simulink model "LQR_v9_two_separate_gyros_discrete"  (R2017b)
settings: Solver=VariableStepAuto  StartTime=0.0  StopTime=10  FixedStep=0.005  RelTol=1e-3
values from neighbouring files (symbols this model uses):
  A = [0 0 0 1 0 0 ... (first row only)    [LQR_PLACE_v9_sep_gryos.m]
  B = [0 0 ... (first row only)    [LQR_PLACE_v9_sep_gryos.m]
  C = [1 0 0 0 0 0 ... (first row only)    [LQR_PLACE_v9_sep_gryos.m]
  Dist_period = 10    [LQR_PLACE_v9_sep_gryos.m]
  F_d = 0    [LQR_PLACE_v9_sep_gryos.m]
  Fd = 300    [LQR_PLACE_v9_sep_gryos.m]
  Init_cond = [ roll_angle, precession_angle1, precession_angle2, roll_rate,     precession_rate1, precession_rate2 ]    [LQR_PLACE_v9_sep_gryos.m]
  Ts = Ts_min    [LQR_PLACE_v9_sep_gryos.m]
  V = [0 ... (first row only)    [LQR_PLACE_v9_sep_gryos.m]
  W = [0 ... (first row only)    [LQR_PLACE_v9_sep_gryos.m]
undefined symbols (not defined in the file or in its folder): Kd
libraries: simulink_extras x3
settings Model: Creator=dbrun  LastModifiedBy=daniel
settings DataIOCC: ReturnWorkspaceOutputs=on
settings SFSimCC: SimUseLocalCustomCode=on
settings RTWCC: RTWUseLocalCustomCode=on

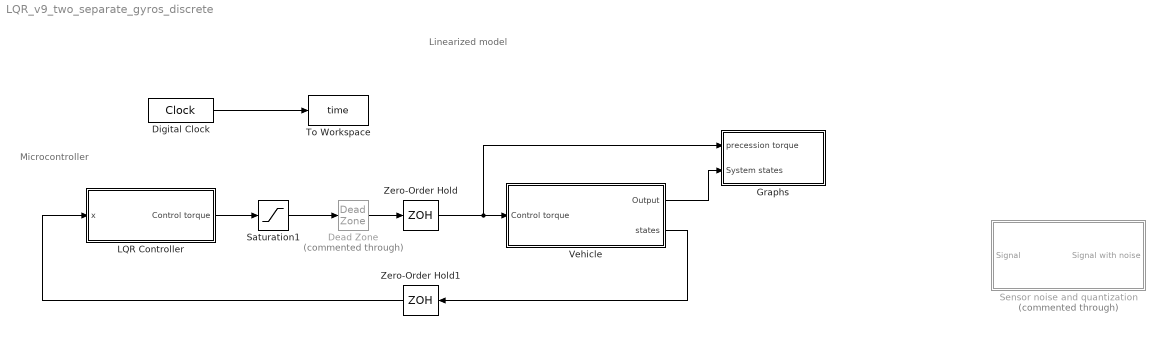
== system LQR_v9_two_separate_gyros_discrete ==
  note: Linearized model
  note: Microcontroller
  Dead Zone : DeadZone  Commented=through  LowerValue=-4  UpperValue=4  SaturateOnIntegerOverflow=on
  Digital Clock : DigitalClock  SampleTime=Ts
  Graphs : Subsystem
  "LQR Controller " : Subsystem
  Saturation1 : Saturate  UpperLimit=70  LowerLimit=-70
  "Sensor noise and quantization " : Subsystem  Commented=through
  To Workspace : ToWorkspace  VariableName=time  SampleTime=Ts
  "Vehicle " : Subsystem
  Zero-Order Hold : ZeroOrderHold  SampleTime=Ts
  Zero-Order Hold1 : ZeroOrderHold  SampleTime=Ts
  wires:
  "Vehicle "/1("Output ") -> Graphs/2(System states)
  Zero-Order Hold/1 -> Graphs/1(precession torque), "Vehicle "/1(Control torque)
  Zero-Order Hold1/1 -> "LQR Controller "/1(x)
  "LQR Controller "/1(Control torque) -> Saturation1/1
  Dead Zone/1 -> Zero-Order Hold/1
  Digital Clock/1 -> To Workspace/1
  Saturation1/1 -> Dead Zone/1
  "Vehicle "/2("states ") -> Zero-Order Hold1/1

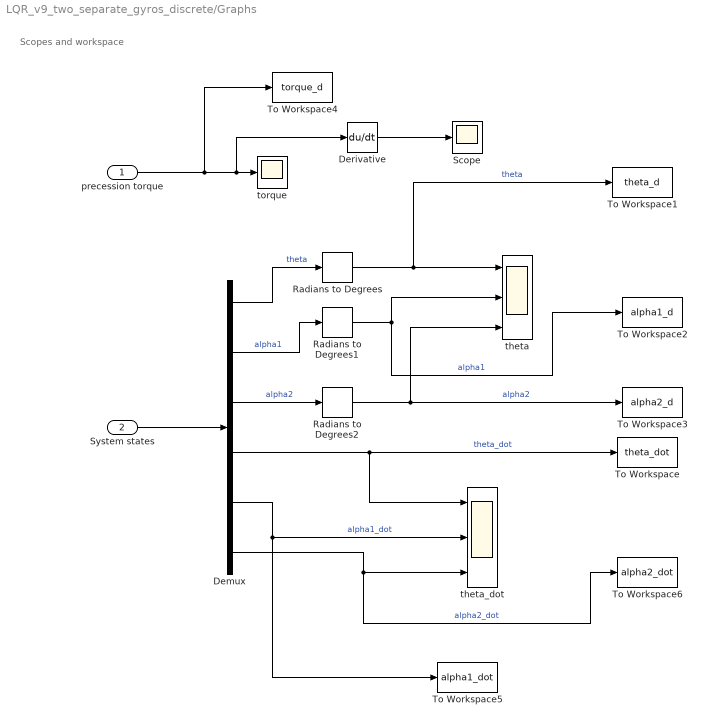
== system LQR_v9_two_separate_gyros_discrete/Graphs ==
  note: Scopes and workspace
  precession torque : Inport
  System states : Inport  Port=2
  Demux : Demux  Outputs=6
  Derivative : Derivative
  Radians to Degrees : simulink_extras/Transformations/Radians to Degrees
  Radians to Degrees1 : simulink_extras/Transformations/Radians to Degrees
  Radians to Degrees2 : simulink_extras/Transformations/Radians to Degrees
  Scope : Scope
  To Workspace : ToWorkspace  VariableName=theta_dot  SampleTime=-1
  To Workspace1 : ToWorkspace  VariableName=theta_d  SampleTime=-1
  To Workspace2 : ToWorkspace  VariableName=alpha1_d  SampleTime=-1
  To Workspace3 : ToWorkspace  VariableName=alpha2_d  SampleTime=-1
  To Workspace4 : ToWorkspace  VariableName=torque_d  SampleTime=-1
  To Workspace5 : ToWorkspace  VariableName=alpha1_dot  SampleTime=-1
  To Workspace6 : ToWorkspace  VariableName=alpha2_dot  SampleTime=-1
  theta : Scope  NumInputPorts=3
  theta_dot : Scope  NumInputPorts=3
  torque : Scope
  wires:
  System states/1 -> Demux/1
  Demux/1 -> Radians to Degrees/1  "theta"
  Demux/2 -> Radians to Degrees1/1  "alpha1"
  Demux/3 -> Radians to Degrees2/1  "alpha2"
  Demux/4 -> theta_dot/1, To Workspace/1  "theta_dot"
  Demux/5 -> To Workspace5/1, theta_dot/2  "alpha1_dot"
  Demux/6 -> To Workspace6/1, theta_dot/3  "alpha2_dot"
  Radians to Degrees1/1 -> theta/2, To Workspace2/1  "alpha1"
  Radians to Degrees/1 -> To Workspace1/1, theta/1  "theta"
  Radians to Degrees2/1 -> To Workspace3/1, theta/3  "alpha2"
  precession torque/1 -> To Workspace4/1, Derivative/1, torque/1
  Derivative/1 -> Scope/1

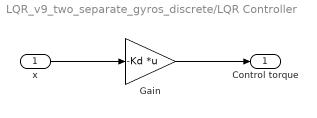
== system LQR_v9_two_separate_gyros_discrete/LQR Controller  ==
  x : Inport  SampleTime=Ts
  Gain : Gain  Gain=-Kd  Multiplication=Matrix(K*u)
  Control torque : Outport  SampleTime=Ts
  wires:
  x/1 -> Gain/1
  Gain/1 -> Control torque/1

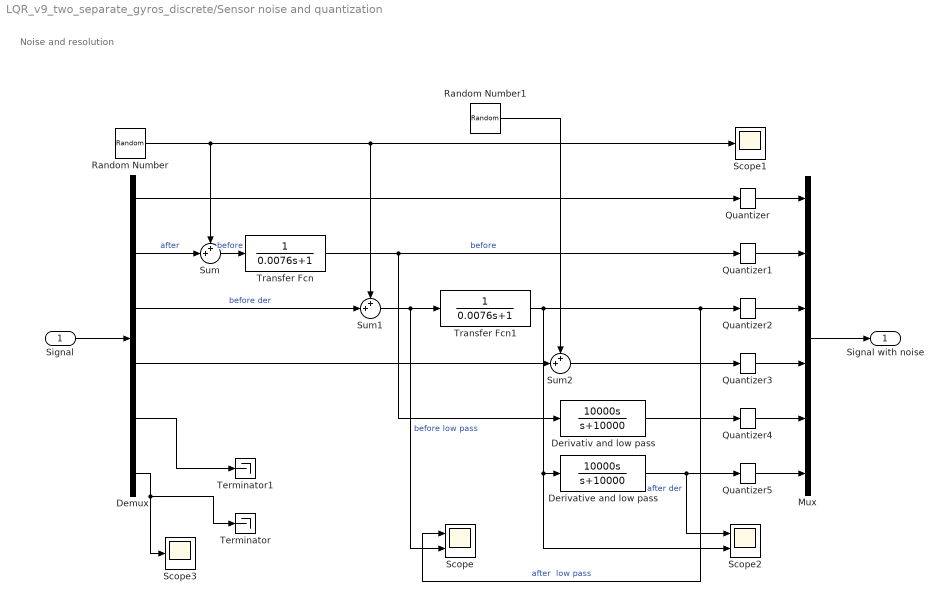
== system LQR_v9_two_separate_gyros_discrete/Sensor noise and quantization  ==
  note: Noise and resolution
  "Signal " : Inport
  Demux : Demux  Outputs=6
  "Derivativ and low pass " : TransferFcn  Numerator=[10000 0]  Denominator=[1 10000]
  "Derivative and low pass " : TransferFcn  Numerator=[10000 0]  Denominator=[1 10000]
  Mux : Mux  Inputs=6
  Quantizer : Quantizer  QuantizationInterval=imu_quant_ang
  Quantizer1 : Quantizer  QuantizationInterval=enc_quant_ang
  Quantizer2 : Quantizer  QuantizationInterval=enc_quant_ang
  Quantizer3 : Quantizer  QuantizationInterval=imu_quant_vel
  Quantizer4 : Quantizer  QuantizationInterval=enc_quant_vel
  Quantizer5 : Quantizer  QuantizationInterval=imu_quant_vel
  Random Number : RandomNumber  Variance=0.00005  Seed=2345  SampleTime=0.3
  Random Number1 : RandomNumber  Variance=0.00005  Seed=2345  SampleTime=0.3
  Scope : Scope  NumInputPorts=2
  Scope1 : Scope
  Scope2 : Scope  NumInputPorts=2
  Scope3 : Scope
  Sum : Sum  Inputs=++|
  Sum1 : Sum  Inputs=++|
  Sum2 : Sum  Inputs=++|
  Terminator : Terminator
  Terminator1 : Terminator
  Transfer Fcn : TransferFcn  Denominator=[0.0076 1]
  Transfer Fcn1 : TransferFcn  Denominator=[0.0076 1]
  "Signal with noise " : Outport
  wires:
  Quantizer1/1 -> Mux/2
  Random Number/1 -> Scope1/1, Sum1/1, Sum/1
  Quantizer2/1 -> Mux/3
  Quantizer4/1 -> Mux/5
  Quantizer/1 -> Mux/1
  "Signal "/1 -> Demux/1
  Quantizer5/1 -> Mux/6
  Demux/1 -> Quantizer/1
  Quantizer3/1 -> Mux/4
  Mux/1 -> "Signal with noise "/1
  Demux/2 -> Sum/2  "after"
  Sum/1 -> Transfer Fcn/1  "before"
  Demux/3 -> Sum1/2  "before der"
  Sum1/1 -> Scope/2, Transfer Fcn1/1  "before low pass"
  Transfer Fcn/1 -> "Derivativ and low pass "/1, Quantizer1/1  "before"
  Transfer Fcn1/1 -> Scope2/2, "Derivative and low pass "/1, Quantizer2/1, Scope/1  "after  low pass"
  Sum2/1 -> Quantizer3/1
  Demux/4 -> Sum2/2
  Demux/6 -> Scope3/1, Terminator/1
  Demux/5 -> Terminator1/1
  Random Number1/1 -> Sum2/1
  "Derivativ and low pass "/1 -> Quantizer4/1
  "Derivative and low pass "/1 -> Scope2/1, Quantizer5/1  "after der"

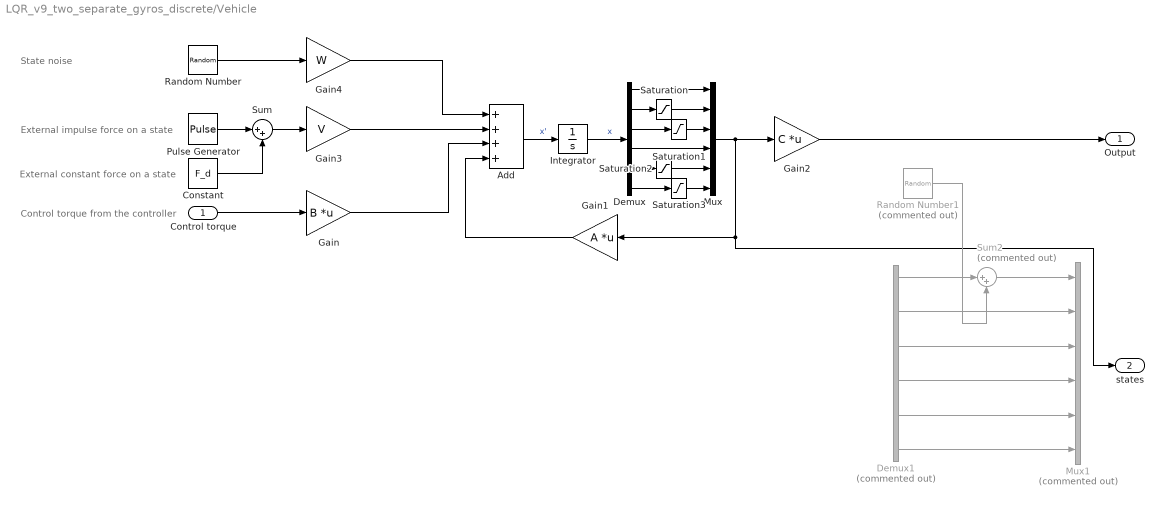
== system LQR_v9_two_separate_gyros_discrete/Vehicle  ==
  note: External constant force on a state
  note: Control torque from the controller
  note: External impulse force on a state
  note: State noise
  Control torque : Inport  SampleTime=Ts
  Add : Sum  Inputs=++++
  Constant : Constant  Value=F_d
  Demux : Demux  Outputs=6
  Demux1 : Demux  Commented=on  Outputs=6
  Gain : Gain  Gain=B  Multiplication=Matrix(K*u)
  Gain1 : Gain  Gain=A  Multiplication=Matrix(K*u)
  Gain2 : Gain  Gain=C  Multiplication=Matrix(K*u)
  Gain3 : Gain  Gain=V
  Gain4 : Gain  Gain=W
  Integrator : Integrator  InitialCondition=Init_cond
  Mux : Mux  Inputs=6
  Mux1 : Mux  Commented=on  Inputs=6
  Pulse Generator : DiscretePulseGenerator  PulseType=Time based  Amplitude=Fd  Period=Dist_period  PulseWidth=5  PhaseDelay=5
  Random Number : RandomNumber  Variance=0.01  Seed=34567  SampleTime=Ts
  Random Number1 : RandomNumber  Commented=on  Variance=0.00001  Seed=23456  SampleTime=Ts
  Saturation : Saturate  UpperLimit=(80*pi)/180  LowerLimit=-(80*pi)/180
  Saturation1 : Saturate  UpperLimit=(80*pi)/180  LowerLimit=-(80*pi)/180
  Saturation2 : Saturate  UpperLimit=4.1  LowerLimit=-4.1
  Saturation3 : Saturate  UpperLimit=4.1  LowerLimit=-4.1
  Sum : Sum  Inputs=|++
  Sum2 : Sum  Commented=on  Inputs=|++
  "Output " : Outport  SampleTime=Ts
  "states " : Outport  Port=2  SampleTime=Ts
  wires:
  Add/1 -> Integrator/1  "x'"
  Gain/1 -> Add/3
  Control torque/1 -> Gain/1
  Gain2/1 -> "Output "/1
  Random Number/1 -> Gain4/1
  Gain1/1 -> Add/4
  Gain3/1 -> Add/2
  Pulse Generator/1 -> Sum/1
  Sum/1 -> Gain3/1
  Constant/1 -> Sum/2
  Gain4/1 -> Add/1
  Demux/3 -> Saturation1/1
  Demux/6 -> Saturation3/1
  Saturation1/1 -> Mux/3
  Demux/2 -> Saturation/1
  Demux/5 -> Saturation2/1
  Demux/4 -> Mux/4
  Saturation/1 -> Mux/2
  Demux/1 -> Mux/1
  Integrator/1 -> Demux/1  "x"
  Mux/1 -> "states "/1, Gain1/1, Gain2/1
  Saturation2/1 -> Mux/5
  Saturation3/1 -> Mux/6
  Demux1/1 -> Sum2/1
  Sum2/1 -> Mux1/1
  Demux1/3 -> Mux1/3
  Demux1/2 -> Mux1/2
  Demux1/4 -> Mux1/4
  Random Number1/1 -> Sum2/2
  Demux1/6 -> Mux1/6
  Demux1/5 -> Mux1/5
